simulink model "linearize_simulink"  (R2025a)
settings: Solver=VariableStepAuto  StartTime=0.0  StopTime=10.0  RelTol=1e-3
values from neighbouring files (symbols this model uses):
  K = 1.75e-4    (= 0.000175)    [system_id.m]
undefined symbols (not defined in the file or in its folder): den, num
settings Model: Creator=USER  LastModifiedBy=USER

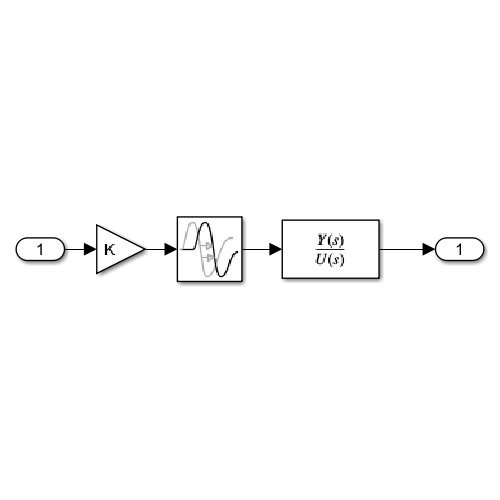
[thumbnail: Simulink's stored preview of the top-level diagram]
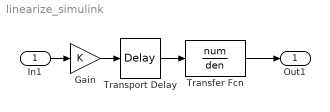
== system linearize_simulink ==
  In1 : Inport
  Gain : Gain  Gain=K
  Transfer Fcn : TransferFcn  Numerator=num  Denominator=den
  Transport Delay : TransportDelay  DelayTime=9.3  PadeOrder=4
  Out1 : Outport
  wires:
  In1/1 -> Gain/1
  Transfer Fcn/1 -> Out1/1
  Gain/1 -> Transport Delay/1
  Transport Delay/1 -> Transfer Fcn/1
